simulink model "Controller_Stabilization_Simul_Final"  (R2025a)
settings: Solver=ode4  StartTime=Tstart  StopTime=Tend  FixedStep=Tsim  RelTol=1e-3
values from neighbouring files (symbols this model uses):
  Kg = 1/0.00067    (= 1492.53731343)    [Controller_Stabilization_Design.m]    (also in Controller_Stabilization_Pole_Placement.m; Controller_Stabilization_Simulation.m)
  Ki = (wn^2 /(Km * Kg * Pm))    [Controller_Stabilization_Design.m]    (also in Controller_Stabilization_Pole_Placement.m; Controller_Stabilization_Simulation.m = 0.0776073069853)
  Kp = ((2 * wn * zeta / Pm) - 1) / (Km * Kg)    [Controller_Stabilization_Design.m]    (also in Controller_Stabilization_Pole_Placement.m; Controller_Stabilization_Simulation.m = 0.00117352840074)
  Ts = 0.005    [Controller_Stabilization_Simulation.m]
  Tsim = 0.001    [Controller_Stabilization_Simulation.m]
settings Model: Creator=Ryuminseo  LastModifiedBy=Ryuminseo

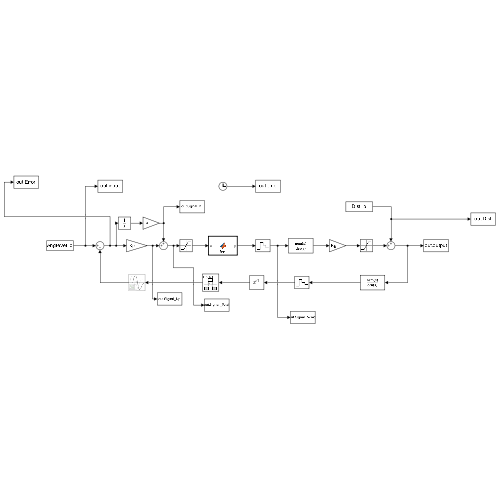
[thumbnail: Simulink's stored preview of the top-level diagram]
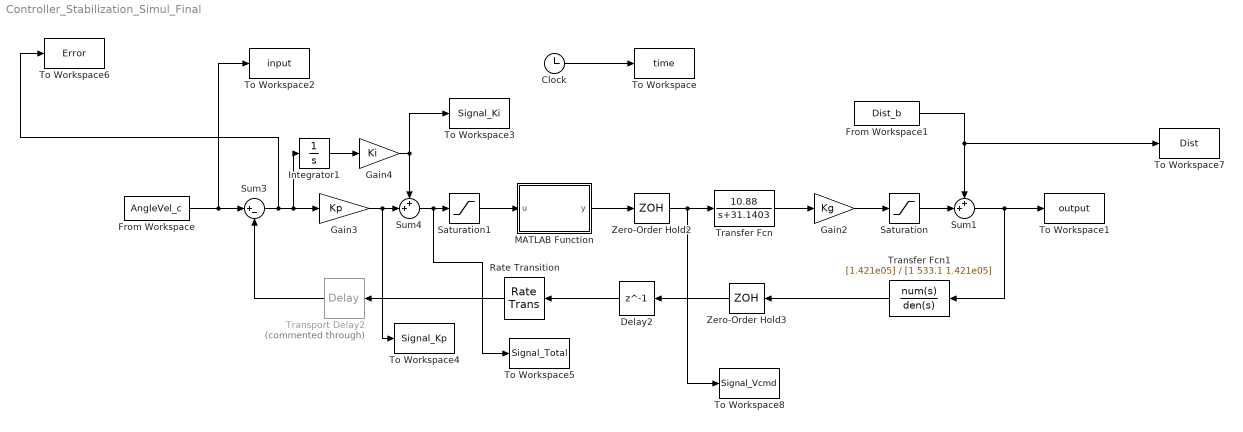
== system Controller_Stabilization_Simul_Final ==
  Clock : Clock
  Delay2 : Delay  DelayLength=1  InitialCondition=0  SampleTime=Ts
  From Workspace : FromWorkspace  VariableName=AngleVel_c  SampleTime=-1
  From Workspace1 : FromWorkspace  VariableName=Dist_b  SampleTime=Ts
  Gain2 : Gain  Gain=Kg
  Gain3 : Gain  Gain=Kp
  Gain4 : Gain  Gain=Ki
  Integrator1 : Integrator
  MATLAB Function : MATLAB Function  TreatAsAtomicUnit=on
  Rate Transition : RateTransition  Deterministic=off
  Saturation : Saturate  UpperLimit=1200  LowerLimit=-1200
  Saturation1 : Saturate  UpperLimit=2.5  LowerLimit=-2.5
  Sum1 : Sum  Inputs=++|
  Sum3 : Sum  Inputs=|+-
  Sum4 : Sum  Inputs=++|
  To Workspace : ToWorkspace  VariableName=time  SampleTime=-1
  To Workspace1 : ToWorkspace  VariableName=output  SampleTime=Tsim
  To Workspace2 : ToWorkspace  VariableName=input  SampleTime=-1
  To Workspace3 : ToWorkspace  VariableName=Signal_Ki  SampleTime=-1
  To Workspace4 : ToWorkspace  VariableName=Signal_Kp  SampleTime=-1
  To Workspace5 : ToWorkspace  VariableName=Signal_Total  SampleTime=-1
  To Workspace6 : ToWorkspace  VariableName=Error  SampleTime=-1
  To Workspace7 : ToWorkspace  VariableName=Dist  SampleTime=Ts
  To Workspace8 : ToWorkspace  VariableName=Signal_Vcmd  SampleTime=Ts
  Transfer Fcn : TransferFcn  Numerator=[10.88]  Denominator=[1 31.1403]
  Transfer Fcn1 : TransferFcn  Numerator=[1.421e05]  Denominator=[1 533.1 1.421e05]
  Transport Delay2 : TransportDelay  Commented=through  DelayTime=Ts
  Zero-Order Hold2 : ZeroOrderHold  SampleTime=Ts
  Zero-Order Hold3 : ZeroOrderHold  SampleTime=Ts
  wires:
  Transfer Fcn/1 -> Gain2/1
  Clock/1 -> To Workspace/1
  Gain2/1 -> Saturation/1
  Saturation1/1 -> MATLAB Function/1(u)
  Sum3/1 -> To Workspace6/1, Gain3/1, Integrator1/1
  Delay2/1 -> Rate Transition/1
  Sum4/1 -> To Workspace5/1, Saturation1/1
  Gain3/1 -> To Workspace4/1, Sum4/2
  Gain4/1 -> Sum4/1, To Workspace3/1
  Integrator1/1 -> Gain4/1
  From Workspace/1 -> To Workspace2/1, Sum3/1
  Saturation/1 -> Sum1/2
  Sum1/1 -> Transfer Fcn1/1, To Workspace1/1
  From Workspace1/1 -> To Workspace7/1, Sum1/1
  Zero-Order Hold3/1 -> Delay2/1
  Zero-Order Hold2/1 -> To Workspace8/1, Transfer Fcn/1
  MATLAB Function/1(y) -> Zero-Order Hold2/1
  Rate Transition/1 -> Transport Delay2/1
  Transport Delay2/1 -> Sum3/2
  Transfer Fcn1/1 -> Zero-Order Hold3/1

== matlab function Controller_Stabilization_Simul_Final/MATLAB Function ==
  data: u input; y output
function y = fcn(u)

    if u >= -0.1 && u <= 0.1
        y = 0;
        
    else
        y = u;
    end
end
